simulink model "simuMFtps"  (R2021a)
settings: Solver=VariableStepAuto  StartTime=0.0  StopTime=1800  RelTol=1e-3
values from neighbouring files (symbols this model uses):
  C = tf( [0.2634 0.0008563], [1 0])    [control_tps.m]    (also in rl_pid_tps.m = Kc*( (s +zero)^2)/(s*(s +paf)); rl_tps.m = Kc*((s+double(zero))/s))
  C2 = (Kp*s + (Kp/Ti))/s    [rl_tps.m]
  P = tf([0  0.02098/0.000325],[1/0.000325 0.000325/0.000325])    [control_tps.m]    (also in rl_pid_tps.m = Ke/(1+s*tau); rl_tps.m = Ke/(1+s*tau))
undefined symbols (not defined in the file or in its folder): C1, H, pi_cd, pif
libraries: simulink x1
settings Model: Creator=jricl  LastModifiedBy=jricl
settings SolverCC: AlgebraicLoopSolver=TrustRegion

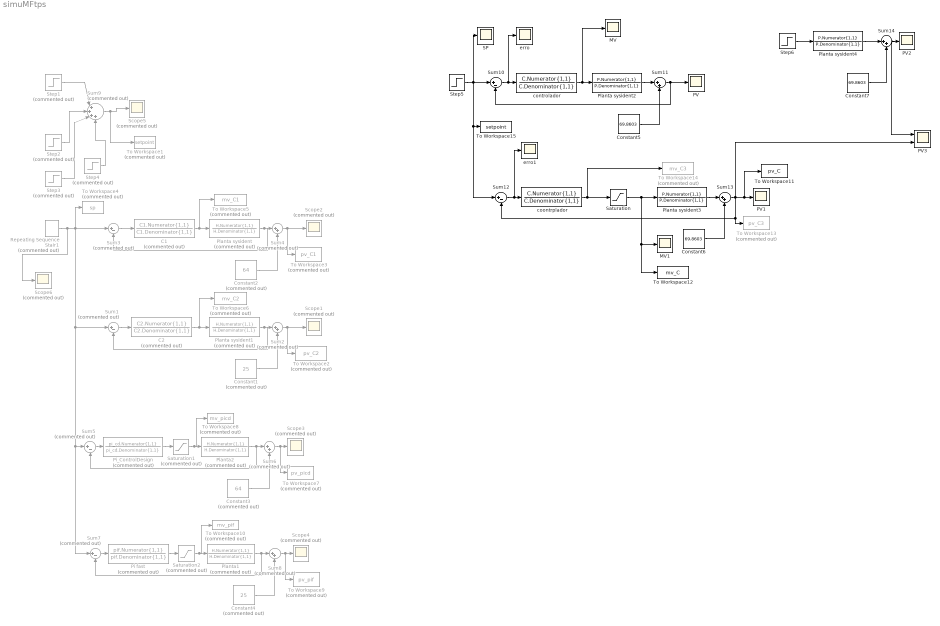
== system simuMFtps ==
  C1 : TransferFcn  Commented=on  Numerator=C1.Numerator{1,1}  Denominator=C1.Denominator{1,1}
  C2 : TransferFcn  Commented=on  Numerator=C2.Numerator{1,1}  Denominator=C2.Denominator{1,1}
  Constant1 : Constant  Commented=on  Value=25
  Constant2 : Constant  Commented=on  Value=64
  Constant3 : Constant  Commented=on  Value=64
  Constant4 : Constant  Commented=on  Value=25
  Constant5 : Constant  Value=69.8603
  Constant6 : Constant  Value=69.8603
  Constant7 : Constant  Value=69.8603
  MV : Scope
  MV1 : Scope
  PV : Scope
  PV1 : Scope
  PV2 : Scope
  PV3 : Scope  NumInputPorts=2
  Pi fast : TransferFcn  Commented=on  Numerator=pif.Numerator{1,1}  Denominator=pif.Denominator{1,1}
  Pi_ControlDesign : TransferFcn  Commented=on  Numerator=pi_cd.Numerator{1,1}  Denominator=pi_cd.Denominator{1,1}
  Planta sysident : TransferFcn  Commented=on  Numerator=H.Numerator{1,1}  Denominator=H.Denominator{1,1}
  Planta sysident1 : TransferFcn  Commented=on  Numerator=H.Numerator{1,1}  Denominator=H.Denominator{1,1}
  Planta sysident2 : TransferFcn  Numerator=P.Numerator{1,1}  Denominator=P.Denominator{1,1}
  Planta sysident3 : TransferFcn  Numerator=P.Numerator{1,1}  Denominator=P.Denominator{1,1}
  Planta sysident4 : TransferFcn  Numerator=P.Numerator{1,1}  Denominator=P.Denominator{1,1}
  Planta1 : TransferFcn  Commented=on  Numerator=H.Numerator{1,1}  Denominator=H.Denominator{1,1}
  Planta2 : TransferFcn  Commented=on  Numerator=H.Numerator{1,1}  Denominator=H.Denominator{1,1}
  Repeating Sequence Stair1 : simulink/Sources/Repeating Sequence Stair  Commented=on  OutValues=[ 69.40-64]  tsamp=1  OutMin=[]  OutMax=[]  OutDataTypeStr=double  OutputDataTypeScalingMode=double  OutDataType=fixdt(0,8)  ConRadixGroup=Best Precision: Vector-wise  OutScaling=2^-12
  SP : Scope
  Saturation : Saturate  UpperLimit=0.31  LowerLimit=0
  Saturation1 : Saturate  Commented=on  UpperLimit=0.320  LowerLimit=0.100
  Saturation2 : Saturate  Commented=on  UpperLimit=100  LowerLimit=0
  Scope{1..6} (6 alike) : Scope  Commented=on
  Step1 : Step  Commented=on  Time=3675  Before=30  After=35
  Step2 : Step  Commented=on  Time=3675*2  After=5
  Step3 : Step  Commented=on  Time=3675*3  After=5
  Step4 : Step  Commented=on  Time=3675*4  After=5
  Step5 : Step  Time=0  Before=69.8603  After=71.16
  Step6 : Step  Time=0  After=0.044
  Sum{1,3,5,7} (4 alike) : Sum  Commented=on  Inputs=|+-
  Sum10 : Sum  Inputs=|+-
  Sum11 : Sum  Inputs=|++
  Sum12 : Sum  Inputs=|+-
  Sum13 : Sum  Inputs=|++
  Sum14 : Sum  Inputs=|++
  Sum{2,4,6,8} (4 alike) : Sum  Commented=on  Inputs=|++
  Sum9 : Sum  Commented=on  Inputs=|++++
  To Workspace1 : ToWorkspace  Commented=on  VariableName=setpoint  SaveFormat=Timeseries  SampleTime=-1
  To Workspace10 : ToWorkspace  Commented=on  VariableName=mv_pif  SaveFormat=Timeseries  SampleTime=-1
  To Workspace11 : ToWorkspace  VariableName=pv_C  SaveFormat=Timeseries  SampleTime=-1
  To Workspace12 : ToWorkspace  VariableName=mv_C  SaveFormat=Timeseries  SampleTime=-1
  To Workspace13 : ToWorkspace  Commented=on  VariableName=pv_C3  SaveFormat=Timeseries  SampleTime=-1
  To Workspace14 : ToWorkspace  Commented=on  VariableName=mv_C3  SaveFormat=Timeseries  SampleTime=-1
  To Workspace15 : ToWorkspace  VariableName=setpoint  SaveFormat=Timeseries  SampleTime=-1
  To Workspace2 : ToWorkspace  Commented=on  VariableName=pv_C2  SaveFormat=Timeseries  SampleTime=-1
  To Workspace3 : ToWorkspace  Commented=on  VariableName=pv_C1  SaveFormat=Timeseries  SampleTime=-1
  To Workspace4 : ToWorkspace  Commented=on  VariableName=sp  SaveFormat=Timeseries  SampleTime=-1
  To Workspace5 : ToWorkspace  Commented=on  VariableName=mv_C1  SaveFormat=Timeseries  SampleTime=-1
  To Workspace6 : ToWorkspace  Commented=on  VariableName=mv_C2  SaveFormat=Timeseries  SampleTime=-1
  To Workspace7 : ToWorkspace  Commented=on  VariableName=pv_picd  SaveFormat=Timeseries  SampleTime=-1
  To Workspace8 : ToWorkspace  Commented=on  VariableName=mv_picd  SaveFormat=Timeseries  SampleTime=-1
  To Workspace9 : ToWorkspace  Commented=on  VariableName=pv_pif  SaveFormat=Timeseries  SampleTime=-1
  controlador : TransferFcn  Numerator=C.Numerator{1,1}  Denominator=C.Denominator{1,1}
  coontrplador : TransferFcn  Numerator=C.Numerator{1,1}  Denominator=C.Denominator{1,1}
  erro : Scope
  erro1 : Scope
  wires:
  Constant2/1 -> Sum4/2
  Sum4/1 -> Scope2/1, To Workspace3/1
  Sum3/1 -> C1/1
  C1/1 -> Planta sysident/1, To Workspace5/1
  Planta sysident/1 -> Sum4/1, Sum3/2
  Step3/1 -> Sum9/3
  Sum9/1 -> To Workspace1/1, Scope5/1
  Step2/1 -> Sum9/2
  Planta sysident1/1 -> Sum1/2, Sum2/1
  C2/1 -> To Workspace6/1, Planta sysident1/1
  Sum1/1 -> C2/1
  Sum2/1 -> To Workspace2/1, Scope1/1
  Constant1/1 -> Sum2/2
  Sum6/1 -> Scope3/1, To Workspace7/1
  Constant3/1 -> Sum6/2
  Planta2/1 -> Sum5/2, Sum6/1
  Saturation1/1 -> To Workspace8/1, Planta2/1
  Sum5/1 -> Pi_ControlDesign/1
  Pi_ControlDesign/1 -> Saturation1/1
  Repeating Sequence Stair1/1 -> Scope6/1, Sum1/1, Sum7/1, Sum5/1, Sum3/1, To Workspace4/1
  Pi fast/1 -> Saturation2/1
  Sum7/1 -> Pi fast/1
  Saturation2/1 -> Planta1/1, To Workspace10/1
  Planta1/1 -> Sum8/1, Sum7/2
  Constant4/1 -> Sum8/2
  Sum8/1 -> To Workspace9/1, Scope4/1
  Step1/1 -> Sum9/1
  Step4/1 -> Sum9/4
  Planta sysident2/1 -> Sum11/1
  controlador/1 -> MV/1, Planta sysident2/1
  Sum10/1 -> erro/1, controlador/1
  Constant5/1 -> Sum11/2
  Sum11/1 -> Sum10/2, PV/1
  Sum13/1 -> To Workspace13/1, Sum12/2, PV3/2, To Workspace11/1, PV1/1
  Step5/1 -> To Workspace15/1, Sum12/1, Sum10/1, SP/1
  Constant6/1 -> Sum13/2
  Sum12/1 -> coontrplador/1, erro1/1
  coontrplador/1 -> Saturation/1, To Workspace14/1
  Planta sysident3/1 -> Sum13/1
  Saturation/1 -> To Workspace12/1, MV1/1, Planta sysident3/1
  Step6/1 -> Planta sysident4/1
  Planta sysident4/1 -> Sum14/1
  Constant7/1 -> Sum14/2
  Sum14/1 -> PV3/1, PV2/1
